simulink model "vC_3ph_MR2"  (Simulink 7.9)
settings: Solver=ode14x  StartTime=0.0  StopTime=20/60  FixedStep=Ts1  RelTol=1e-3
PostLoadFcn:
  | , if any(exist('dsrtsu_mdlpostloadfcn', 'file') == [2, 3, 6]), try dsrtsu_mdlpostloadfcn('Execute', bdroot); catch fprintf('Error in PostLoadFcn (dsrtsu_mdlpostloadfcn) for model "%s":\n %s\n', bdroot, lasterr); end, end,
InitFcn:
  | vC_ini
values from neighbouring files (symbols this model uses):
  C = Cideal+deltaC    (= 4e-05)    [IMC_calculo_limites_thetas.m]    (also in IMC_ini.m; JORGE_controlador_LCL_malha_interna.m; LCL_PAPM.m; R_in_LCL.m)
  excitacao_persistente = 0    [iC_ini.m]    (also in vC_ini.m)
  flag_time = 60/60    (= 1)    [iC_ini.m]    (also in vC_ini.m = 0)
  init_time = 60/60    (= 1)    [iC_ini.m]    (also in vC_ini.m)
  L1 = L1ideal+deltaL1    (= 0.002)    [IMC_calculo_limites_thetas.m]    (also in IMC_ini.m; LCL_PAPM.m; R_in_LCL.m; calculo_FTs.m)
  L2 = L2ideal+deltaL2+Lgideal+deltaLg    (= 0.002)    [IMC_calculo_limites_thetas.m]    (also in IMC_ini.m; LCL_PAPM.m; R_in_LCL.m; calculo_FTs.m)
  param_change_time = 60/60    (= 1)    [iC_ini.m]    (also in vC_ini.m)
  R1 = R1ideal+deltaR1    (= 1)    [IMC_calculo_limites_thetas.m]    (also in IMC_ini.m; R_in_LCL.m = 0; gera_resultados.m = 0; iC_ini.m = 0)
  R2 = R2ideal+deltaR2+Rgideal+deltaRg    (= 1)    [IMC_calculo_limites_thetas.m]    (also in IMC_ini.m; R_in_LCL.m = 0; gera_resultados.m = 0; iC_ini.m = 0)
  R_init = 10    [iC_ini.m]    (also in vC_ini.m)
  ref_phaseInv_time = 60/60    (= 1)    [iC_ini.m]    (also in vC_ini.m)
  ref_step_time = 60/60    (= 1)    [iC_ini.m]    (also in vC_ini.m)
  short_OFF_time = 61/60    (= 1.01666666667)    [vC_ini.m]
  short_ON_time = 60/60    (= 1)    [vC_ini.m]
  Ts = 0.5    [IMC_calculo_limites_thetas.m]    (also in IMC_datta_ini.m; IMC_ini.m = 8.33333333333e-05; JORGE_controlador_LCL_malha_interna.m = 8.33333333333e-05; LCL_PAPM.m = 8.33333333333e-05)
  Ts1 = Ts/10    (= 8.33333333333e-06)    [iC_ini.m]    (also in vC_ini.m)
  VCC = 1700    [iC_ini.m]    (also in vC_ini.m = 1200)
undefined symbols (not defined in the file or in its folder): D1, Delta
libraries: powerlib x38, powerlib_extras x1
(part 1 of 3)
settings Model: DSRTSU_INTERNAL_RTI_VER=390  DSRTSU_INTERNAL_RTI_TYPE=rti1103  Creator=dpbernardon  LastModifiedBy=marcelodurgante  BufferReuse=off
settings SolverCC: AutoInsertRateTranBlk=on
settings OptimizationCC: BlockReduction=off  OptimizeBlockIOStorage=off  BufferReuse=off  ExpressionFolding=off  LocalBlockOutputs=off
settings DebuggingCC: FcnCallInpInsideContextMsg=Use local settings
settings HardwareCC: ProdIntDivRoundTo=Zero  ProdEndianess=BigEndian  ProdHWDeviceType=Generic->Custom  TargetIntDivRoundTo=Zero  TargetEndianess=BigEndian  TargetHWDeviceType=Generic->Custom
settings RTWCC: SystemTargetFile=rti1103.tlc  MakeCommand=make_rti  TemplateMakefile=rti1103.tmf  Description=dSPACE DS1103 Hardware Platform  ProcessScript=rti1103_make_rtw_hook
settings STFCustomTargetCC: CodeReplacementLibrary=ANSI_C  ParMdlRefBuildCompliant=on  GeneratePreprocessorConditionals=Disable all  MatFileLogging=on  SystemTargetFile=rti1103.tlc
settings GRTTargetCC: CompOptLevelCompliant=off  ConcurrentExecutionCompliant=off  CombineOutputUpdateFcns=off  GRTInterface=on  ExtModeMexFile=noextcomm
settings CustomProperty: DataType=RTWOptions_EnumType_C__dSPACE RCPHIL 72_matlab_rti1103_tlc_rti1103_1InitialSimState  Value=RUN
settings EnumStrPairs: String=RUN

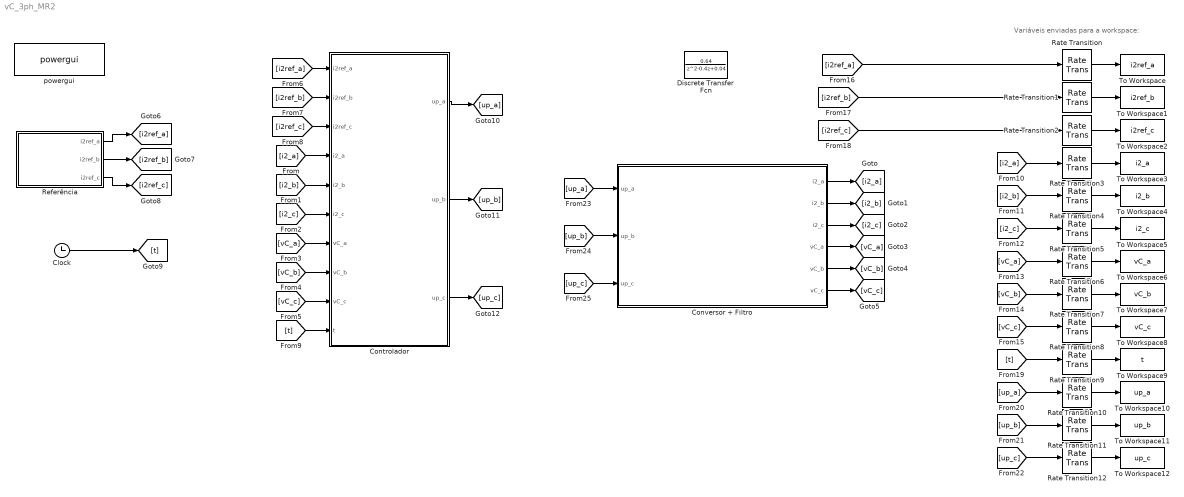
== system vC_3ph_MR2 ==
  note: Variáveis enviadas para a workspace:
  Clock : Clock
  Controlador : Subsystem
  Conversor + Filtro : Subsystem
  Discrete Transfer Fcn : DiscreteTransferFcn  Numerator=[0 0.64]  Denominator=[1 -0.4 0.04]  SampleTime=Ts
  Rate Transition{,1..12} (13 alike) : RateTransition  OutPortSampleTime=Ts1
  Referência : Subsystem
  To Workspace : ToWorkspace  VariableName=i2ref_a  SampleTime=Ts1
  To Workspace1 : ToWorkspace  VariableName=i2ref_b  SampleTime=Ts1
  To Workspace10 : ToWorkspace  VariableName=up_a  SampleTime=Ts1
  To Workspace11 : ToWorkspace  VariableName=up_b  SampleTime=Ts1
  To Workspace12 : ToWorkspace  VariableName=up_c  SampleTime=Ts1
  To Workspace2 : ToWorkspace  VariableName=i2ref_c  SampleTime=Ts1
  To Workspace3 : ToWorkspace  VariableName=i2_a  SampleTime=Ts1
  To Workspace4 : ToWorkspace  VariableName=i2_b  SampleTime=Ts1
  To Workspace5 : ToWorkspace  VariableName=i2_c  SampleTime=Ts1
  To Workspace6 : ToWorkspace  VariableName=vC_a  SampleTime=Ts1
  To Workspace7 : ToWorkspace  VariableName=vC_b  SampleTime=Ts1
  To Workspace8 : ToWorkspace  VariableName=vC_c  SampleTime=Ts1
  To Workspace9 : ToWorkspace  VariableName=t  SampleTime=Ts1
  powergui : powerlib/powergui  Priority=1  SimulationMode=Discrete  SolverType=Tustin  SampleTime=Ts1  frequency=60  SPID=off  DisableSnubberDevices=off  DisableRonSwitches=off  DisableVfSwitches=off  SwTol=0  Interpol=off  DisplayEquations=off  FunctionMessages=off  frequencyindice=0  Pbase=100e6  ErrMax=1e-4  Iterations=50  UnitsV=kV  UnitsW=MW  echomessages=off  HookPort=off  EnableUseOfTLC=off  x0status=blocks  RestoreLinks=warning  ResistiveCurrentMeasurement=off  Frange=[0:2:500]  Ylog=off  Xlog=on  ShowGrid=off  save=off  variable=ZData  ZoomFFT=off  StartTime=0.0  cycles=1  DisplayStyle=1  fundamental=60  FreqAxis=off  MaxFrequency=1000  frequencyindicesteady=1  RmsSteady=1  display=off  Ts=0  methode=off
  wires:
  [i2_a] -> Controlador/4(i2_a)
  [i2_b] -> Controlador/5(i2_b)
  [i2_c] -> Controlador/6(i2_c)
  [vC_a] -> Controlador/7(vC_a)
  [vC_b] -> Controlador/8(vC_b)
  [vC_c] -> Controlador/9(vC_c)
  Referência/2(i2ref_b) -> [i2ref_b]
  Referência/1(i2ref_a) -> [i2ref_a]
  Referência/3(i2ref_c) -> [i2ref_c]
  [i2ref_a] -> Controlador/1(i2ref_a)
  [i2ref_b] -> Controlador/2(i2ref_b)
  [i2ref_c] -> Controlador/3(i2ref_c)
  Clock/1 -> [t]
  [t] -> Controlador/10(t)
  [i2_a] -> Rate Transition3/1
  [i2_b] -> Rate Transition4/1
  [i2_c] -> Rate Transition5/1
  [vC_a] -> Rate Transition6/1
  [vC_b] -> Rate Transition7/1
  [vC_c] -> Rate Transition8/1
  [t] -> Rate Transition9/1
  Rate Transition/1 -> To Workspace/1
  Rate Transition1/1 -> To Workspace1/1
  Rate Transition2/1 -> To Workspace2/1
  Rate Transition3/1 -> To Workspace3/1
  Rate Transition4/1 -> To Workspace4/1
  Rate Transition5/1 -> To Workspace5/1
  Rate Transition6/1 -> To Workspace6/1
  Rate Transition7/1 -> To Workspace7/1
  Rate Transition8/1 -> To Workspace8/1
  Rate Transition9/1 -> To Workspace9/1
  [up_a] -> Rate Transition10/1
  [up_b] -> Rate Transition11/1
  [up_c] -> Rate Transition12/1
  Rate Transition10/1 -> To Workspace10/1
  Rate Transition11/1 -> To Workspace11/1
  Rate Transition12/1 -> To Workspace12/1
  Controlador/1(up_a) -> [up_a]
  Controlador/2(up_b) -> [up_b]
  Controlador/3(up_c) -> [up_c]
  [up_a] -> Conversor + Filtro/1(up_a)
  [up_b] -> Conversor + Filtro/2(up_b)
  [up_c] -> Conversor + Filtro/3(up_c)
  Conversor + Filtro/1(i2_a) -> [i2_a]
  Conversor + Filtro/2(i2_b) -> [i2_b]
  Conversor + Filtro/3(i2_c) -> [i2_c]
  Conversor + Filtro/4(vC_a) -> [vC_a]
  Conversor + Filtro/5(vC_b) -> [vC_b]
  Conversor + Filtro/6(vC_c) -> [vC_c]
  [i2ref_a] -> Rate Transition/1
  [i2ref_b] -> Rate Transition1/1
  [i2ref_c] -> Rate Transition2/1

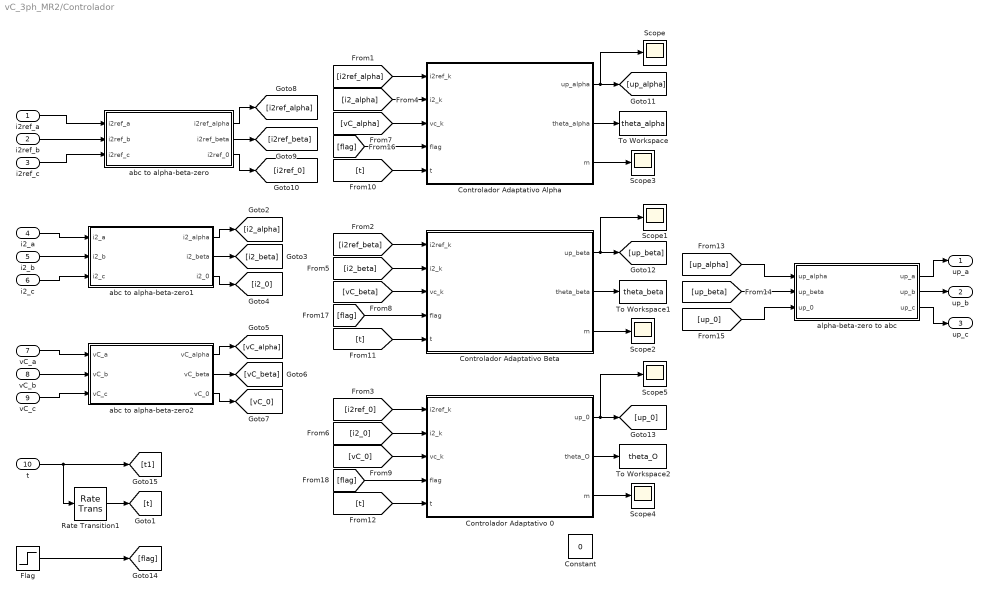
== system vC_3ph_MR2/Controlador ==
  i2ref_a : Inport
  i2ref_b : Inport  Port=2
  i2ref_c : Inport  Port=3
  i2_a : Inport  Port=4
  i2_b : Inport  Port=5
  i2_c : Inport  Port=6
  vC_a : Inport  Port=7
  vC_b : Inport  Port=8
  vC_c : Inport  Port=9
  t : Inport  Port=10
  Constant : Constant  Value=0  SampleTime=Ts
  Controlador Adaptativo 0 : MATLAB Function  TreatAsAtomicUnit=on  SystemSampleTime=Ts
      settings: MinAlgLoopOccurrences=on  RTWSystemCode=Function
  Controlador Adaptativo Alpha : MATLAB Function  TreatAsAtomicUnit=on  SystemSampleTime=Ts
      settings: MinAlgLoopOccurrences=on  RTWSystemCode=Function
  Controlador Adaptativo Beta : MATLAB Function  TreatAsAtomicUnit=on  SystemSampleTime=Ts
      settings: MinAlgLoopOccurrences=on  RTWSystemCode=Function
  Flag : Step  Time=flag_time  Before=1  After=0  SampleTime=Ts
  Rate Transition1 : RateTransition  OutPortSampleTime=Ts
  Scope{,1..5} (6 alike) : Scope
      Scope settings: YMin=-5500  YMax=5000  SaveName=ScopeData3
      Scope1 settings: YMin=-5500  YMax=5000  SaveName=ScopeData4
      Scope2 settings: YMin=-5500  YMax=5000  SaveName=ScopeData5
      Scope3 settings: YMin=-5500  YMax=5000
      Scope4 settings: YMin=-5500  YMax=5000
      Scope5 settings: YMin=-5500  YMax=5000  SaveName=ScopeData2
  To Workspace : ToWorkspace  VariableName=theta_alpha  SampleTime=Ts1
  To Workspace1 : ToWorkspace  VariableName=theta_beta  SampleTime=Ts1
  To Workspace2 : ToWorkspace  VariableName=theta_O  SampleTime=Ts1
  abc to alpha-beta-zero : MATLAB Function  TreatAsAtomicUnit=on
  abc to alpha-beta-zero1 : MATLAB Function  TreatAsAtomicUnit=on
  abc to alpha-beta-zero2 : MATLAB Function  TreatAsAtomicUnit=on
  alpha-beta-zero to abc : MATLAB Function  TreatAsAtomicUnit=on  SystemSampleTime=Ts
  up_a : Outport
  up_b : Outport  Port=2
  up_c : Outport  Port=3
  wires:
  i2ref_a/1 -> abc to alpha-beta-zero/1(i2ref_a)
  i2ref_b/1 -> abc to alpha-beta-zero/2(i2ref_b)
  i2ref_c/1 -> abc to alpha-beta-zero/3(i2ref_c)
  t/1 -> Rate Transition1/1, [t1]
  Rate Transition1/1 -> [t]
  i2_a/1 -> abc to alpha-beta-zero1/1(i2_a)
  i2_b/1 -> abc to alpha-beta-zero1/2(i2_b)
  i2_c/1 -> abc to alpha-beta-zero1/3(i2_c)
  vC_a/1 -> abc to alpha-beta-zero2/1(vC_a)
  vC_b/1 -> abc to alpha-beta-zero2/2(vC_b)
  vC_c/1 -> abc to alpha-beta-zero2/3(vC_c)
  abc to alpha-beta-zero1/1(i2_alpha) -> [i2_alpha]
  abc to alpha-beta-zero1/2(i2_beta) -> [i2_beta]
  abc to alpha-beta-zero1/3(i2_0) -> [i2_0]
  abc to alpha-beta-zero2/2(vC_beta) -> [vC_beta]
  abc to alpha-beta-zero2/1(vC_alpha) -> [vC_alpha]
  abc to alpha-beta-zero2/3(vC_0) -> [vC_0]
  abc to alpha-beta-zero/1(i2ref_alpha) -> [i2ref_alpha]
  abc to alpha-beta-zero/2(i2ref_beta) -> [i2ref_beta]
  abc to alpha-beta-zero/3(i2ref_0) -> [i2ref_0]
  [i2ref_alpha] -> Controlador Adaptativo Alpha/1(i2ref_k)
  [i2ref_beta] -> Controlador Adaptativo Beta/1(i2ref_k)
  [i2ref_0] -> Controlador Adaptativo 0/1(i2ref_k)
  [i2_alpha] -> Controlador Adaptativo Alpha/2(i2_k)
  [i2_beta] -> Controlador Adaptativo Beta/2(i2_k)
  [i2_0] -> Controlador Adaptativo 0/2(i2_k)
  [vC_alpha] -> Controlador Adaptativo Alpha/3(vc_k)
  [vC_beta] -> Controlador Adaptativo Beta/3(vc_k)
  [vC_0] -> Controlador Adaptativo 0/3(vc_k)
  [t] -> Controlador Adaptativo 0/5(t)
  [t] -> Controlador Adaptativo Beta/5(t)
  [t] -> Controlador Adaptativo Alpha/5(t)
  Controlador Adaptativo Beta/1(up_beta) -> [up_beta], Scope1/1
  alpha-beta-zero to abc/2(up_b) -> up_b/1
  alpha-beta-zero to abc/3(up_c) -> up_c/1
  alpha-beta-zero to abc/1(up_a) -> up_a/1
  [up_beta] -> alpha-beta-zero to abc/2(up_beta)
  [up_alpha] -> alpha-beta-zero to abc/1(up_alpha)
  [up_0] -> alpha-beta-zero to abc/3(up_0)
  Flag/1 -> [flag]
  [flag] -> Controlador Adaptativo Alpha/4(flag)
  [flag] -> Controlador Adaptativo Beta/4(flag)
  [flag] -> Controlador Adaptativo 0/4(flag)
  Controlador Adaptativo Alpha/2(theta_alpha) -> To Workspace/1
  Controlador Adaptativo Beta/2(theta_beta) -> To Workspace1/1
  Controlador Adaptativo 0/2(theta_O) -> To Workspace2/1
  Controlador Adaptativo Alpha/1(up_alpha) -> [up_alpha], Scope/1
  Controlador Adaptativo Alpha/3(m) -> Scope3/1
  Controlador Adaptativo Beta/3(m) -> Scope2/1
  Controlador Adaptativo 0/1(up_0) -> [up_0], Scope5/1
  Controlador Adaptativo 0/3(m) -> Scope4/1
